simulink model "SP_linsysGet"  (R2016b)
settings: Solver=ode2  StartTime=0.0  StopTime=1  FixedStep=0.02  RelTol=1e-3
StopFcn:
  | A = StateSpace.A.Data(:,:,end);
  | B = StateSpace.B.Data(:,:,end);
  | C = StateSpace.C.Data(:,:,end);
  | if ( size(C,1) == 1 )
  |    D = StateSpace.D.Data(end);
  | else
  |    D = StateSpace.D.Data(:,:,end);
  | end
  | 
  | save linsys.mat A B C D;
undefined symbols (not defined in the file or in its folder): op
libraries: aerolibatmos2 x1
settings Model: Creator=whn  LastModifiedBy=whn
settings DataIOCC: SaveFormat=StructureWithTime
settings OptimizationCC: LifeSpan=inf
settings DebuggingCC: SFExecutionAtInitializationDiag=none
settings HardwareCC: ProdBitPerSizeT=32  ProdBitPerPtrDiffT=32  ProdWordSize=32  ProdHWDeviceType=Specified
settings ConfigComp: CovSFcnEnable=off

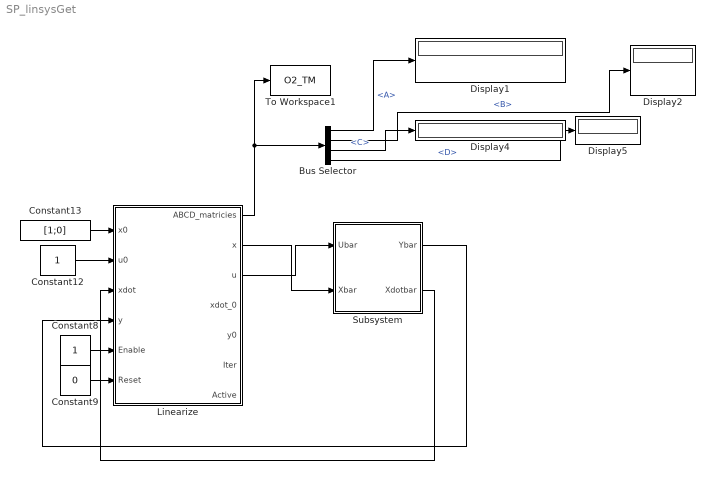
== system SP_linsysGet ==
  Bus Selector : BusSelector  OutputSignals=A,B,C,D
  Constant12 : Constant  VectorParams1D=off
  Constant13 : Constant  Value=[1;0]  VectorParams1D=off
  Constant8 : Constant
  Constant9 : Constant  Value=0
  Display{1..2,4..5} (4 alike) : Display
  Linearize : Subsystem  TreatAsAtomicUnit=on  mask(T-MATS: Linearize Library Block){N_XPer_M=[0.001 0.001], N_UPer_M=0.001, N_Y_M=1}
      mask prompts: N_XPer_M "N_XPer_M - x Perturbation values (mx1)"; N_UPer_M "N_UPer_M - u Perturbation values (nx1)"; N_Y_M "N_Y_M - Number of expected y values (1x1)"
      mask help:
      | Determine State-space equation for a given system where:
      |
      | (xdot - xdot_0) = A*(x - x0) + B*(u - u0)
      | (y - y0) = C*(x - x0) + D*(u - u0)
      |
      | During operation each plant state (x) and input (u) will be set to an initial condition then perturbed separately. Perturbed inputs and system effects are compared against the baseline to determine the A,B,C, and D matricies. Perturbation sized are specified below. x0, u0, xdot_0, and y0 values are initial conditions.
      | Matrix sizes are specified as:
      | xdot and x : mx1
      | y : px1
      | u : nx1
      | A : mxm
      | B : mxn
      | C : pxm
      | D : pxn
      mask Help: web(which('Solver_TMATS_Linearize.html'),'-helpbrowser')
  Subsystem : Subsystem
  To Workspace1 : ToWorkspace  VariableName=O2_TM  SaveFormat=Timeseries  SampleTime=-1
  wires:
  Constant8/1 -> Linearize/5(Enable)
  Constant9/1 -> Linearize/6(Reset)
  Constant12/1 -> Linearize/2(u0)
  Constant13/1 -> Linearize/1(x0)
  Bus Selector/1 -> Display1/1  "<A>"
  Bus Selector/2 -> Display2/1  "<B>"
  Bus Selector/3 -> Display4/1  "<C>"
  Bus Selector/4 -> Display5/1  "<D>"
  Linearize/1(ABCD_matricies) -> Bus Selector/1, To Workspace1/1
  Linearize/3(u) -> Subsystem/1(Ubar)
  Subsystem/1(Ybar) -> Linearize/4(y)
  Subsystem/2(Xdotbar) -> Linearize/3(xdot)
  Linearize/2(x) -> Subsystem/2(Xbar)

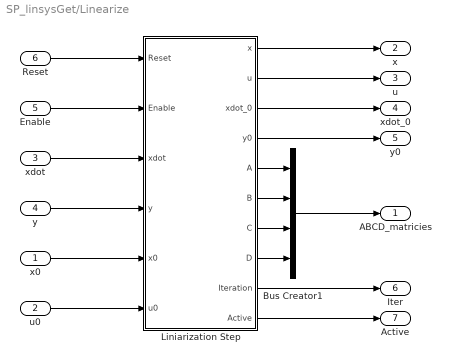
== system SP_linsysGet/Linearize ==
  x0 : Inport
  u0 : Inport  Port=2
  xdot : Inport  Port=3
  y : Inport  Port=4
  Enable : Inport  Port=5
  Reset : Inport  Port=6
  Bus Creator1 : BusCreator  Inputs=4
  Liniarization Step : Subsystem  TreatAsAtomicUnit=on
  ABCD_matricies : Outport
  x : Outport  Port=2
  u : Outport  Port=3
  xdot_0 : Outport  Port=4
  y0 : Outport  Port=5
  Iter : Outport  Port=6
  Active : Outport  Port=7
  wires:
  Enable/1 -> Liniarization Step/2(Enable)
  xdot/1 -> Liniarization Step/3(xdot)
  Bus Creator1/1 -> ABCD_matricies/1
  Reset/1 -> Liniarization Step/1(Reset)
  Liniarization Step/1(x) -> x/1
  Liniarization Step/2("u ") -> u/1
  Liniarization Step/5(A) -> Bus Creator1/1
  Liniarization Step/6(B) -> Bus Creator1/2
  Liniarization Step/7(C) -> Bus Creator1/3
  Liniarization Step/8(D) -> Bus Creator1/4
  y/1 -> Liniarization Step/4(y)
  x0/1 -> Liniarization Step/5(x0)
  u0/1 -> Liniarization Step/6(u0)
  Liniarization Step/9(Iteration) -> Iter/1
  Liniarization Step/10(Active) -> Active/1
  Liniarization Step/3(xdot_0) -> xdot_0/1
  Liniarization Step/4(y0) -> y0/1

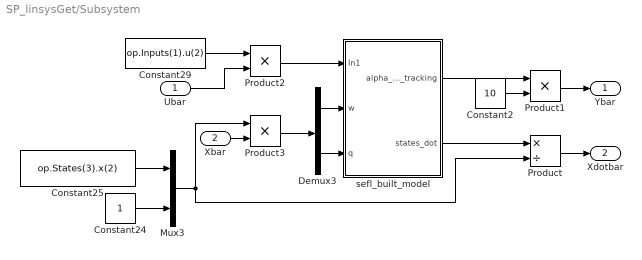
== system SP_linsysGet/Subsystem ==
  Ubar : Inport
  Xbar : Inport  Port=2
  Constant2 : Constant  Value=10
  Constant24 : Constant
  Constant25 : Constant  Value=op.States(3).x(2)
  Constant29 : Constant  Value=op.Inputs(1).u(2)
  Demux3 : Demux  Outputs=2
  Mux3 : Mux  Inputs=2
  Product : Product  Inputs=*/
  Product1 : Product
  Product2 : Product
  Product3 : Product
  sefl_built_model : Subsystem
  Ybar : Outport
  Xdotbar : Outport  Port=2
  wires:
  Mux3/1 -> Product/2, Product3/1
  Xbar/1 -> Product3/2
  sefl_built_model/1(alpha_for_tracking) -> Product1/1
  Product1/1 -> Ybar/1
  Product3/1 -> Demux3/1
  sefl_built_model/2(states_dot) -> Product/1
  Constant29/1 -> Product2/1
  Constant2/1 -> Product1/2
  Product2/1 -> sefl_built_model/1(In1)
  Product/1 -> Xdotbar/1
  Demux3/1 -> sefl_built_model/2(w)
  Constant25/1 -> Mux3/1
  Constant24/1 -> Mux3/2
  Demux3/2 -> sefl_built_model/3(q)
  Ubar/1 -> Product2/2

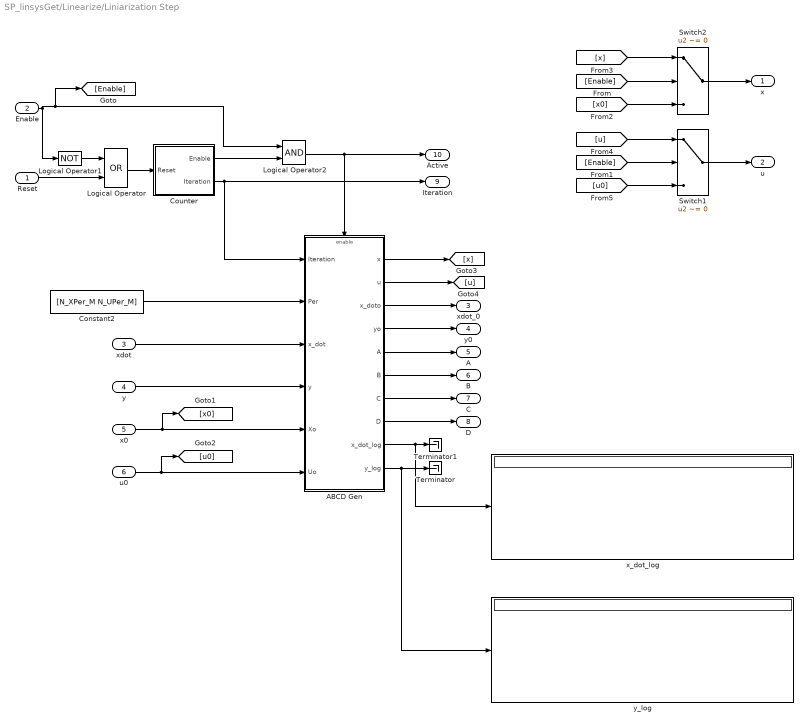
== system SP_linsysGet/Linearize/Liniarization Step ==
  Reset : Inport
  Enable : Inport  Port=2
  xdot : Inport  Port=3
  y : Inport  Port=4
  x0 : Inport  Port=5
  u0 : Inport  Port=6
  ABCD Gen : Subsystem
  Constant2 : Constant  Value=[N_XPer_M N_UPer_M]
  Counter : Subsystem  mask{N_Ind_M=length(N_XPer_M) + length(N_UPer_M)}
      mask prompts: N_Ind_M "number of independents, N_Ind_M"
  Logical Operator : Logic  Operator=OR  AllPortsSameDT=off  OutDataTypeStr=boolean
  Logical Operator1 : Logic  Operator=NOT  AllPortsSameDT=off  OutDataTypeStr=boolean
  Logical Operator2 : Logic  AllPortsSameDT=off  OutDataTypeStr=boolean
  Switch1 : Switch  Criteria=u2 ~= 0
  Switch2 : Switch  Criteria=u2 ~= 0
  Terminator : Terminator
  Terminator1 : Terminator
  x_dot_log : Display
  y_log : Display
  x : Outport
  "u " : Outport  Port=2
  xdot_0 : Outport  Port=3
  y0 : Outport  Port=4
  A : Outport  Port=5
  B : Outport  Port=6
  C : Outport  Port=7
  D : Outport  Port=8
  Iteration : Outport  Port=9
  Active : Outport  Port=10
  wires:
  [x] -> Switch2/1
  [x0] -> Switch2/3
  [u0] -> Switch1/3
  [u] -> Switch1/1
  Switch1/1 -> "u "/1
  Switch2/1 -> x/1
  [Enable] -> Switch1/2
  [Enable] -> Switch2/2
  Enable/1 -> Logical Operator1/1, Logical Operator2/1, [Enable]
  Counter/1(Enable) -> Logical Operator2/2
  Logical Operator1/1 -> Logical Operator/1
  Logical Operator/1 -> Counter/1(Reset)
  ABCD Gen/7(C) -> C/1
  ABCD Gen/8(D) -> D/1
  Counter/2(Iteration) -> ABCD Gen/1(Iteration), Iteration/1
  x0/1 -> ABCD Gen/5(Xo), [x0]
  Logical Operator2/1 -> Active/1, ABCD Gen/Enable
  Reset/1 -> Logical Operator/2
  ABCD Gen/1(x) -> [x]
  Constant2/1 -> ABCD Gen/2(Per)
  xdot/1 -> ABCD Gen/3(x_dot)
  u0/1 -> ABCD Gen/6(Uo), [u0]
  y/1 -> ABCD Gen/4(y)
  ABCD Gen/10(y_log) -> y_log/1, Terminator/1
  ABCD Gen/9(x_dot_log) -> x_dot_log/1, Terminator1/1
  ABCD Gen/2(u) -> [u]
  ABCD Gen/5(A) -> A/1
  ABCD Gen/6(B) -> B/1
  ABCD Gen/3(x_doto) -> xdot_0/1
  ABCD Gen/4(yo) -> y0/1

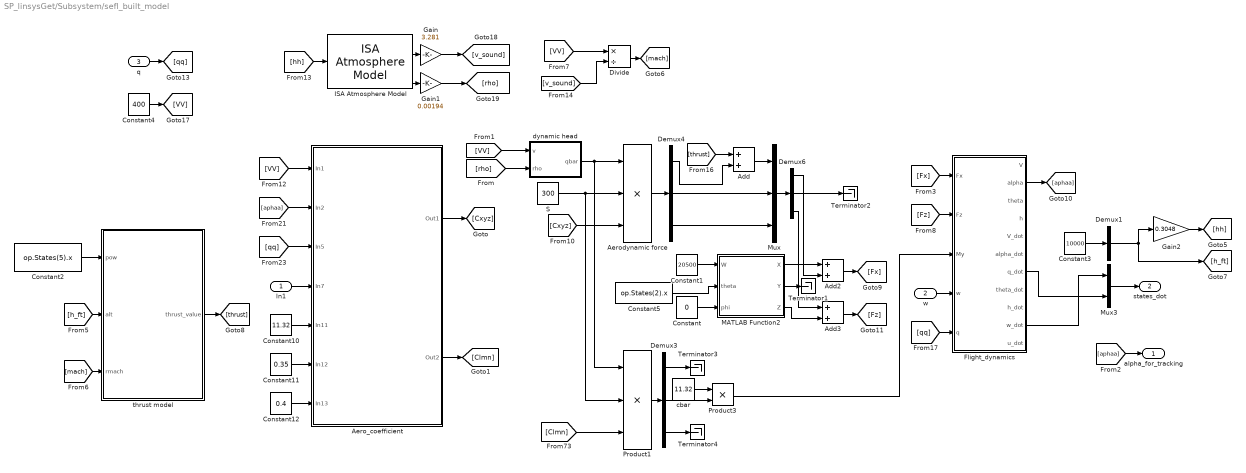
== system SP_linsysGet/Subsystem/sefl_built_model ==
  In1 : Inport
  w : Inport  Port=2
  q : Inport  Port=3
  Add : Sum
  Add2 : Sum
  Add3 : Sum
  Aero_coefficient : Subsystem
      mask Display:
      | port_label('input', 1, 'vt')
      | port_label('input', 2, 'alpha')
      | 
      | port_label('input', 3, 'q')
      | 
      | port_label('input', 4, 'el')
      | 
      | 
      | 
      | port_label('input', 5, 'cbar')
      | port_label('input', 6, 'xcgr')
      | port_label('input', 7, 'xcg')
      | port_label('output', 1, 'Cxz')
      | port_label('output', 2, 'Cm')
  "Aerodynamic force " : Product  Inputs=3
  Constant : Constant  Value=0
  Constant1 : Constant  Value=20500
  Constant10 : Constant  Value=11.32
  Constant11 : Constant  Value=0.35
  Constant12 : Constant  Value=0.4
  Constant2 : Constant  Value=op.States(5).x
  Constant3 : Constant  Value=10000
  Constant4 : Constant  Value=400
  Constant5 : Constant  Value=op.States(2).x
  Demux1 : Demux  Outputs=1
  Demux3 : Demux  Outputs=3
  Demux4 : Demux  Outputs=3
  Demux6 : Demux  Outputs=3
  Divide : Product  Inputs=*/
  Flight_dynamics : Subsystem
  Gain : Gain  Gain=3.281
  Gain1 : Gain  Gain=0.00194
  Gain2 : Gain  Gain=0.3048
  ISA Atmosphere Model : aerolibatmos2/ISA Atmosphere Model  custom=off  g=9.80665  gamma=1.4  R=287.0531  L=0.0065  h_trop=11000  h_strat=20000  rho0=1.225  P0=101325  T0=288.15  h0=0
  MATLAB Function2 : MATLAB Function  TreatAsAtomicUnit=on
  Mux : Mux  Inputs=3
  Mux3 : Mux  Inputs=2
  Product1 : Product  Inputs=3
  Product3 : Product
  S : Constant  Value=300
  Terminator{1..4} (4 alike) : Terminator
  cbar : Constant  Value=11.32
  dynamic head : MATLAB Function  TreatAsAtomicUnit=on
  thrust model : MATLAB Function  TreatAsAtomicUnit=on
  alpha_for_tracking : Outport
  states_dot : Outport  Port=2
  wires:
  Flight_dynamics/2(alpha) -> [aphaa]
  Mux3/1 -> states_dot/1
  Product3/1 -> Flight_dynamics/3(My)
  [Fz] -> Flight_dynamics/2(Fz)
  [Fx] -> Flight_dynamics/1(Fx)
  Add3/1 -> [Fz]
  Add2/1 -> [Fx]
  MATLAB Function2/2(Y) -> Terminator1/1
  MATLAB Function2/3(Z) -> Add3/2
  Demux6/1 -> Add2/2
  MATLAB Function2/1(X) -> Add2/1
  Constant/1 -> MATLAB Function2/3(phi)
  Constant5/1 -> MATLAB Function2/2(theta)
  Constant1/1 -> MATLAB Function2/1(W)
  Demux6/2 -> Terminator2/1
  Demux6/3 -> Add3/1
  cbar/1 -> Product3/1
  Demux3/2 -> Product3/2
  Product1/1 -> Demux3/1
  [Clmn] -> Product1/3
  S/1 -> Product1/2, "Aerodynamic force "/2
  [Cxyz] -> "Aerodynamic force "/3
  "Aerodynamic force "/1 -> Demux4/1
  [thrust] -> Add/1
  [mach] -> thrust model/3(rmach)
  [h_ft] -> thrust model/2(alt)
  thrust model/1(thrust_value) -> [thrust]
  Gain2/1 -> [hh]
  Constant12/1 -> Aero_coefficient/7(In13)
  Mux/1 -> Demux6/1
  Demux4/1 -> Add/2
  [v_sound] -> Divide/2
  Demux4/2 -> Mux/2
  Add/1 -> Mux/1
  Divide/1 -> [mach]
  Gain/1 -> [v_sound]
  Demux4/3 -> Mux/3
  [hh] -> ISA Atmosphere Model/1
  Demux1/1 -> [h_ft], Gain2/1
  Aero_coefficient/2(Out2) -> [Clmn]
  [rho] -> dynamic head/2(rho)
  Aero_coefficient/1(Out1) -> [Cxyz]
  [VV] -> dynamic head/1(v)
  [VV] -> Divide/1
  Gain1/1 -> [rho]
  Constant11/1 -> Aero_coefficient/6(In12)
  Constant10/1 -> Aero_coefficient/5(In11)
  In1/1 -> Aero_coefficient/4(In7)
  dynamic head/1(qbar) -> "Aerodynamic force "/1, Product1/1
  ISA Atmosphere Model/2 -> Gain/1
  ISA Atmosphere Model/4 -> Gain1/1
  [VV] -> Aero_coefficient/1(In1)
  [aphaa] -> Aero_coefficient/2(In2)
  [qq] -> Aero_coefficient/3(In5)
  q/1 -> [qq]
  Flight_dynamics/10(w_dot) -> Mux3/1
  Flight_dynamics/7(q_dot) -> Mux3/2
  Constant2/1 -> thrust model/1(pow)
  Constant3/1 -> Demux1/1
  Constant4/1 -> [VV]
  [aphaa] -> alpha_for_tracking/1
  w/1 -> Flight_dynamics/4(w)
  [qq] -> Flight_dynamics/5(q)
  Demux3/1 -> Terminator3/1
  Demux3/3 -> Terminator4/1

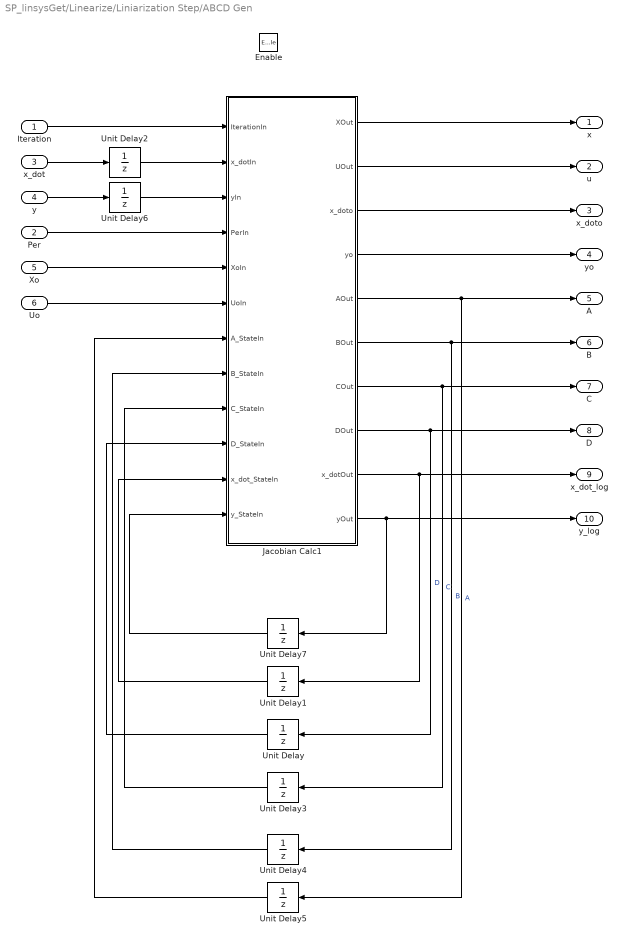
== system SP_linsysGet/Linearize/Liniarization Step/ABCD Gen ==
  Iteration : Inport
  Per : Inport  Port=2
  x_dot : Inport  Port=3
  y : Inport  Port=4
  Xo : Inport  Port=5
  Uo : Inport  Port=6
  Enable : EnablePort
  Jacobian Calc1 : MATLAB Function  TreatAsAtomicUnit=on
  Unit Delay : UnitDelay  InitialCondition=zeros(N_Y_M,length(N_UPer_M))  SampleTime=-1
  Unit Delay1 : UnitDelay  InitialCondition=zeros(length(N_XPer_M),length(N_XPer_M)+length(N_UPer_M)+1)  SampleTime=-1
  Unit Delay2 : UnitDelay  InitialCondition=zeros(length(N_XPer_M),1)  SampleTime=-1
  Unit Delay3 : UnitDelay  InitialCondition=zeros(N_Y_M,length(N_XPer_M))  SampleTime=-1
  Unit Delay4 : UnitDelay  InitialCondition=zeros(length(N_XPer_M),length(N_UPer_M))  SampleTime=-1
  Unit Delay5 : UnitDelay  InitialCondition=zeros(length(N_XPer_M),length(N_XPer_M))  SampleTime=-1
  Unit Delay6 : UnitDelay  InitialCondition=zeros(length(N_Y_M),1)  SampleTime=-1
  Unit Delay7 : UnitDelay  InitialCondition=zeros(N_Y_M,length(N_XPer_M)+length(N_UPer_M)+1)  SampleTime=-1
  x : Outport
  u : Outport  Port=2
  x_doto : Outport  Port=3
  yo : Outport  Port=4
  A : Outport  Port=5
  B : Outport  Port=6
  C : Outport  Port=7
  D : Outport  Port=8
  x_dot_log : Outport  Port=9
  y_log : Outport  Port=10
  wires:
  Unit Delay2/1 -> Jacobian Calc1/2(x_dotIn)
  x_dot/1 -> Unit Delay2/1
  Unit Delay1/1 -> Jacobian Calc1/11(x_dot_StateIn)
  Jacobian Calc1/9(x_dotOut) -> Unit Delay1/1, x_dot_log/1
  Jacobian Calc1/8(DOut) -> Unit Delay/1, D/1  "D"
  Jacobian Calc1/7(COut) -> Unit Delay3/1, C/1  "C"
  Iteration/1 -> Jacobian Calc1/1(IterationIn)
  Per/1 -> Jacobian Calc1/4(PerIn)
  Xo/1 -> Jacobian Calc1/5(XoIn)
  Jacobian Calc1/1(XOut) -> x/1
  Jacobian Calc1/6(BOut) -> Unit Delay4/1, B/1  "B"
  Jacobian Calc1/5(AOut) -> Unit Delay5/1, A/1  "A"
  Unit Delay/1 -> Jacobian Calc1/10(D_StateIn)
  Unit Delay3/1 -> Jacobian Calc1/9(C_StateIn)
  Unit Delay4/1 -> Jacobian Calc1/8(B_StateIn)
  Unit Delay5/1 -> Jacobian Calc1/7(A_StateIn)
  Uo/1 -> Jacobian Calc1/6(UoIn)
  Jacobian Calc1/2(UOut) -> u/1
  Jacobian Calc1/10(yOut) -> Unit Delay7/1, y_log/1
  Unit Delay6/1 -> Jacobian Calc1/3(yIn)
  y/1 -> Unit Delay6/1
  Unit Delay7/1 -> Jacobian Calc1/12(y_StateIn)
  Jacobian Calc1/3(x_doto) -> x_doto/1
  Jacobian Calc1/4(yo) -> yo/1

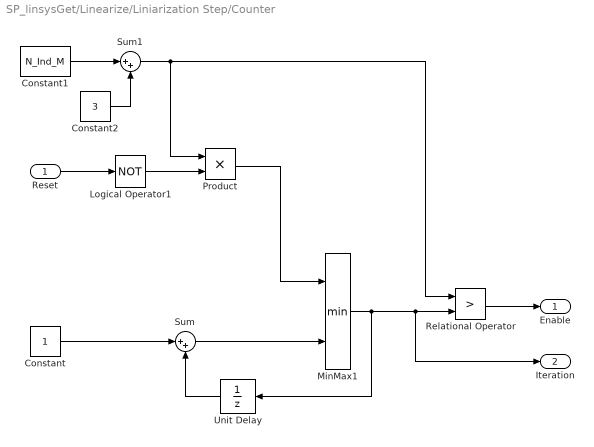
== system SP_linsysGet/Linearize/Liniarization Step/Counter ==
  Reset : Inport
  Constant : Constant
  Constant1 : Constant  Value=N_Ind_M
  Constant2 : Constant  Value=3
  Logical Operator1 : Logic  Operator=NOT  AllPortsSameDT=off  OutDataTypeStr=boolean
  MinMax1 : MinMax  Inputs=2
  Product : Product  RndMeth=Zero
  Relational Operator : RelationalOperator  Operator=>  OutDataTypeStr=boolean  RndMeth=Nearest
  Sum : Sum  Inputs=|++
  Sum1 : Sum  Inputs=|++
  Unit Delay : UnitDelay  SampleTime=-1
  Enable : Outport
  Iteration : Outport  Port=2
  wires:
  Constant1/1 -> Sum1/1
  Constant2/1 -> Sum1/2
  Sum1/1 -> Product/1, Relational Operator/1
  Reset/1 -> Logical Operator1/1
  Logical Operator1/1 -> Product/2
  Relational Operator/1 -> Enable/1
  MinMax1/1 -> Relational Operator/2, Iteration/1, Unit Delay/1
  Unit Delay/1 -> Sum/2
  Sum/1 -> MinMax1/2
  Product/1 -> MinMax1/1
  Constant/1 -> Sum/1

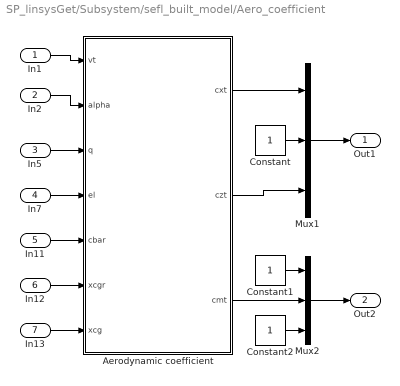
== system SP_linsysGet/Subsystem/sefl_built_model/Aero_coefficient ==
  In1 : Inport
  In2 : Inport  Port=2
  In5 : Inport  Port=3
  In7 : Inport  Port=4
  In11 : Inport  Port=5
  In12 : Inport  Port=6
  In13 : Inport  Port=7
  Aerodynamic coefficient : MATLAB Function  TreatAsAtomicUnit=on
  Constant : Constant
  Constant1 : Constant
  Constant2 : Constant
  Mux1 : Mux  Inputs=3
  Mux2 : Mux  Inputs=3
  Out1 : Outport
  Out2 : Outport  Port=2
  wires:
  Constant2/1 -> Mux2/3
  Constant1/1 -> Mux2/1
  Constant/1 -> Mux1/2
  Mux2/1 -> Out2/1
  Mux1/1 -> Out1/1
  Aerodynamic coefficient/1(cxt) -> Mux1/1
  In13/1 -> Aerodynamic coefficient/7(xcg)
  Aerodynamic coefficient/2(czt) -> Mux1/3
  In12/1 -> Aerodynamic coefficient/6(xcgr)
  In11/1 -> Aerodynamic coefficient/5(cbar)
  Aerodynamic coefficient/3(cmt) -> Mux2/2
  In7/1 -> Aerodynamic coefficient/4(el)
  In2/1 -> Aerodynamic coefficient/2(alpha)
  In1/1 -> Aerodynamic coefficient/1(vt)
  In5/1 -> Aerodynamic coefficient/3(q)

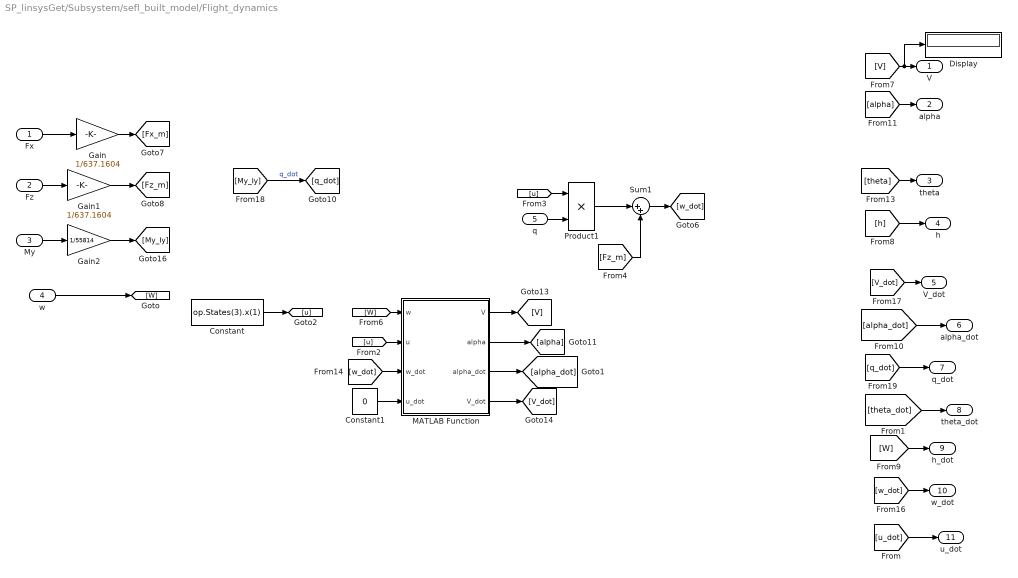
== system SP_linsysGet/Subsystem/sefl_built_model/Flight_dynamics ==
  Fx : Inport
  Fz : Inport  Port=2
  My : Inport  Port=3
  w : Inport  Port=4
  q : Inport  Port=5
  Constant : Constant  Value=op.States(3).x(1)
  Constant1 : Constant  Value=0
  Display : Display
  Gain : Gain  Gain=1/637.1604
  Gain1 : Gain  Gain=1/637.1604
  Gain2 : Gain  Gain=1/55814
  MATLAB Function : MATLAB Function  TreatAsAtomicUnit=on
  Product1 : Product
  Sum1 : Sum  Inputs=|++
  V : Outport
  alpha : Outport  Port=2
  theta : Outport  Port=3
  h : Outport  Port=4
  V_dot : Outport  Port=5
  alpha_dot : Outport  Port=6
  q_dot : Outport  Port=7
  theta_dot : Outport  Port=8
  h_dot : Outport  Port=9
  w_dot : Outport  Port=10
  u_dot : Outport  Port=11
  wires:
  [u_dot] -> u_dot/1
  [w_dot] -> w_dot/1
  [u] -> MATLAB Function/2(u)
  [W] -> h_dot/1
  [h] -> h/1
  MATLAB Function/4(V_dot) -> [V_dot]
  MATLAB Function/1(V) -> [V]
  [theta_dot] -> theta_dot/1
  [q_dot] -> q_dot/1
  [alpha_dot] -> alpha_dot/1
  [V_dot] -> V_dot/1
  [theta] -> theta/1
  [alpha] -> alpha/1
  [V] -> V/1, Display/1
  MATLAB Function/3(alpha_dot) -> [alpha_dot]
  [w_dot] -> MATLAB Function/3(w_dot)
  MATLAB Function/2(alpha) -> [alpha]
  [W] -> MATLAB Function/1(w)
  [My_Iy] -> [q_dot]  "q_dot"
  Sum1/1 -> [w_dot]
  [Fz_m] -> Sum1/2
  Product1/1 -> Sum1/1
  Gain2/1 -> [My_Iy]
  My/1 -> Gain2/1
  Gain1/1 -> [Fz_m]
  Gain/1 -> [Fx_m]
  Fz/1 -> Gain1/1
  Fx/1 -> Gain/1
  Constant/1 -> [u]
  Constant1/1 -> MATLAB Function/4(u_dot)
  [u] -> Product1/1
  w/1 -> [W]
  q/1 -> Product1/2

== matlab function SP_linsysGet/Linearize/Liniarization Step/ABCD Gen/Jacobian Calc1 ==
  data: IterationIn input; XOut output; x_dotIn input; yIn input; PerIn input; XoIn input; UoIn input; A_StateIn input size=[length(N_XPer_M) length(N_XPer_M)]; B_StateIn input size=[length(N_XPer_M) length(N_UPer_M)]; C_StateIn input size=[N_Y_M length(N_XPer_M)]; D_StateIn input size=[N_Y_M length(N_UPer_M)]; x_dot_StateIn input; UOut output; x_doto output; yo output; AOut output; BOut output; COut output size=[N_Y_M length(N_XPer_M)]; DOut output; x_dotOut output; yOut output; y_StateIn input size=[N_Y_M,length(N_XPer_M)+length(N_UPer_M)+1]
function [ XOut, UOut, x_doto, yo, AOut, BOut, COut, DOut, x_dotOut, yOut ] = fcn ...
( IterationIn, x_dotIn, yIn, PerIn, XoIn, UoIn, A_StateIn, B_StateIn, C_StateIn, D_StateIn, x_dot_StateIn, y_StateIn )

% Set inital condiations
i = IterationIn;
XOut = XoIn;
UOut = UoIn;
AOut = A_StateIn;
BOut = B_StateIn;
COut = C_StateIn;
DOut = D_StateIn;
x_dotOut = x_dot_StateIn;
yOut = y_StateIn;

x_doto = x_dot_StateIn(:,1);
yo = y_StateIn(:,1);

% Begin taking data from f(x) at iteration a+1
a = 1;
% Begin determining Jacobian at iteration b+1
b = a+1;
c = a+length(XoIn);
d = c+1;

% Set X&U Output
if i > a && i <= length(XoIn) + a
    XOut(i-a) = XOut(i-a) + PerIn(i - a);
elseif i > c && i <= length(UoIn) + c
    UOut(i-c) = UOut(i-c) + PerIn(i - a);
end

% setup state feedback
if i > a && i<= length(XoIn) + length(UoIn) + a+1;
        x_dotOut(:,i - a) = x_dotIn;
        yOut(:,i - a) = yIn;
end

% Create Jacobian
if i > b && i <= length(XoIn) + b
    if length(XoIn) == 1
        AOut = (x_dotIn - x_dotOut(:,1))/PerIn(1);
        COut = (yIn - yOut(:,1))/PerIn(1);
    else
        AOut(:,i - b) = (x_dotIn - x_dotOut(:,1))/PerIn(i - b);
        COut(:,i - b) = (yIn - yOut(:,1))/PerIn(i - b);
    end
end
if i > d && i <= length(UoIn) + d
    if length(UoIn) == 1
        BOut = (x_dotIn - x_dotOut(:,1))/PerIn(c);
        DOut = (yIn - yOut(:,1))/PerIn(c);
    else
        BOut(:,i - d) = (x_dotIn - x_dotOut(:,1))/PerIn(i - d);
        DOut(:,i - d) = (yIn - yOut(:,1))/PerIn(i - d);
    end
end

== matlab function SP_linsysGet/Subsystem/sefl_built_model/Aero_coefficient/Aerodynamic coefficient ==
  data: vt input; alpha input; q input; cxt output; el input; czt output; cmt output; cbar input; xcgr input; xcg input
function [cxt,czt,cmt]=fcn(vt,alpha,q,el,cbar,xcgr,xcg)
%% ---- Look-up tables and component biuldup ------------
beta=0;
rtod = 180 / pi;
alpha=alpha*rtod;
beta=beta*rtod;
% el=el*rtod;
% ail=ail*rtod;
% rdr=rdr*rtod;
cxt = cx ( alpha, el );
%cyt = cy ( beta, ail, rdr );
czt = cz ( alpha, beta, el );
%dail = ail / 20.0;
%drdr = rdr / 30.0;
%dlda_value = dlda( alpha, beta );
%dldr_value = dldr( alpha, beta );
%clt = cl( alpha, beta ) + dlda_value * dail + dldr_value * drdr;
cmt = cm( alpha, el );
%dnda_value = dnda( alpha, beta );
%dndr_value = dndr( alpha, beta );
%cnt = cn( alpha, beta ) + dnda_value * dail + dndr_value * drdr;

%% ---- Add damping derivatives ------------
tvt = 0.5 / vt;
%b2v = b * tvt;
cq = cbar * q * tvt;
d = damping( alpha );
cxt = cxt + cq * d(1);
%cyt = cyt + b2v * ( d(2) * r + d(3) * p );
czt = czt + cq * d(4);
%clt = clt + b2v * ( d(5) * r + d(6) * p );
cmt = cmt + cq * d(7) + czt * ( xcgr - xcg );
%cnt = cnt + b2v * ( d(8)* r + d(9) * p ) - cyt * ( xcgr - xcg ) * cbar / b;

function dlda_value = dlda ( alpha, beta )

A = [ -.041  -.052  -.053  -.056  -.050  -.056  -.082  -.059  -.042  -.038  -.027  -.017;
      -.041  -.053  -.053  -.053  -.050  -.051  -.066  -.043  -.038  -.027  -.023  -.016;
      -.042  -.053  -.052  -.051  -.049  -.049  -.043  -.035  -.026  -.016  -.018  -.014;
      -.040  -.052  -.051  -.052  -.048  -.048  -.042  -.037  -.031  -.026  -.017  -.012;
      -.043  -.049  -.048  -.049  -.043  -.042  -.042  -.036  -.025  -.021  -.016  -.011;
      -.044  -.048  -.048  -.047  -.042  -.041  -.020  -.028  -.013  -.014  -.011  -.010;
      -.043  -.049  -.047  -.045  -.042  -.037  -.003  -.013  -.010  -.003  -.007  -.008 ];
A = A';  
row = 3;
col = 4;

s = 0.2 * alpha;
k = fix ( s );
if ( k <= -2 )
    k = -1;
end
if ( k >= 9 )
    k = 8;
end
da = s -  k ;
l = k + fix ( sign ( da ) * 1.1 );
%%%%%%%%%%%%%%%%%%%%%%%%%%%%%%%%%%
% added as boundary condition
if l < -2
    l = -2;
elseif l > 9
        l = 9;
end
%%%%%%%%%%%%%%%%%%%%%%%%%%%%%%%%%%
s = 0.1 * beta;
m = fix ( s );
if ( m <= -3 )
   m = -2;
end
if ( m >= 3)
   m = 2;
end
db = s -  m ;
n = m + fix ( sign ( db ) * 1.1 );
%%%%%%%%%%%%%%%%%%%%%%%%%%%%%%%%%%
% added as boundary condition
if n < -3
    n = -3;
elseif n > 3
        n = 3;
end
%%%%%%%%%%%%%%%%%%%%%%%%%%%%%%%%%%
%  disp('k+row'); k+row
%  disp('m+col'); m+col
%  disp('n+col'); n+col
%  disp('l+row'); l+row
t = A( k+row, m+col );
u = A( k+row, n+col );
v = t + abs( da ) * ( A( l+row, m+col ) - t );
w = u + abs( da ) * ( A( l+row, n+col ) - u );
dlda_value = v + ( w - v ) * abs( db );

function dldr_value = dldr ( alpha, beta )

A = [ .005  .017  .014  .010  -.005  .009  .019  .005   .000  -.005  -.011  .008;
      .007  .016  .014  .014   .013  .009  .012  .005   .000   .004   .009  .007;
      .013  .013  .011  .012   .011  .009  .008  .005   .000   .005   .003  .005;
      .018  .015  .015  .014   .014  .014  .014  .015   .013   .011   .006  .001;
      .015  .014  .013  .013   .012  .011  .011  .010   .008   .008   .007  .003;
      .021  .011  .010  .011   .010  .009  .008  .010   .006   .005   .000  .001;
      .023  .010  .011  .011   .011  .010  .008  .010   .006   .014   .020  .000 ];
A = A';  
row = 3;
col = 4;

s = 0.2 * alpha;
k = fix ( s );
if ( k <= -2 )
    k = -1;
end
if ( k >= 9 )
    k = 8;
end
da = s -  k ;
l = k + fix ( sign ( da ) * 1.1 );
%%%%%%%%%%%%%%%%%%%%%%%%%%%%%%%%%%
% added as boundary condition
if l < -2
    l = -2;
elseif l > 9
        l = 9;
end
%%%%%%%%%%%%%%%%%%%%%%%%%%%%%%%%%%
s = 0.1 * beta;
m = fix ( s );
if ( m <= -3 )
   m = -2;
end
if ( m >= 3)
   m = 2;
end
db = s -  m ;
n = m + fix ( sign ( db ) * 1.1 );
%%%%%%%%%%%%%%%%%%%%%%%%%%%%%%%%%%
% added as boundary condition
if n < -3
    n = -3;
elseif n > 3
        n = 3;
end
%%%%%%%%%%%%%%%%%%%%%%%%%%%%%%%%%%
t = A( k+row, m+col );
u = A( k+row, n+col );
v = t + abs( da ) * ( A( l+row, m+col ) - t );
w = u + abs( da ) * ( A( l+row, n+col ) - u );
dldr_value = v + ( w - v ) * abs( db );

function dnda_value = dnda ( alpha, beta )

A = [  .001  -.027  -.017  -.013  -.012  -.016   .001   .017   .011  .017   .008  .016
       .002  -.014  -.016  -.016  -.014  -.019  -.021   .002   .012  .016   .015  .011
      -.006  -.008  -.006  -.006  -.005  -.008  -.005   .007   .004  .007   .006  .006
      -.011  -.011  -.010  -.009  -.008  -.006   .000   .004   .007  .010   .004  .010
      -.015  -.015  -.014  -.012  -.011  -.008  -.002   .002   .006  .012   .011  .011
      -.024  -.010  -.004  -.002  -.001   .003   .014   .006  -.001  .004   .004  .006
      -.022   .002  -.003  -.005  -.003  -.001  -.009  -.009  -.001  .003  -.002  .001  ];
A = A';  
row = 3;
col = 4;

s = 0.2 * alpha;
k = fix ( s );
if ( k <= -2 )
    k = -1;
end
if ( k >= 9 )
    k = 8;
end
da = s -  k ;
l = k + fix ( sign ( da ) * 1.1 );
%%%%%%%%%%%%%%%%%%%%%%%%%%%%%%%%%%
% added as boundary condition
if l < -2
    l = -2;
elseif l > 9
        l = 9;
end
%%%%%%%%%%%%%%%%%%%%%%%%%%%%%%%%%%
s = 0.1 * beta;
m = fix ( s );
if ( m <= -3 )
   m = -2;
end
if ( m >= 3)
   m = 2;
end
db = s -  m ;
n = m + fix ( sign ( db ) * 1.1 );
%%%%%%%%%%%%%%%%%%%%%%%%%%%%%%%%%%
% added as boundary condition
if n < -3
    n = -3;
elseif n > 3
        n = 3;
end
%%%%%%%%%%%%%%%%%%%%%%%%%%%%%%%%%%
t = A( k+row, m+col );
u = A( k+row, n+col );
v = t + abs( da ) * ( A( l+row, m+col ) - t );
w = u + abs( da ) * ( A( l+row, n+col ) - u );
dnda_value = v + ( w - v ) * abs( db );

function dndr_value = dndr ( alpha, beta )

A = [ -.018  -.052  -.052  -.052  -.054  -.049  -.059  -.051  -.030  -.037  -.026  -.013;
      -.028  -.051  -.043  -.046  -.045  -.049  -.057  -.052  -.030  -.033  -.030  -.008;
      -.037  -.041  -.038  -.040  -.040  -.038  -.037  -.030  -.027  -.024  -.019  -.013; 
      -.048  -.045  -.045  -.045  -.044  -.045  -.047  -.048  -.049  -.045  -.033  -.016;
      -.043  -.044  -.041  -.041  -.040  -.038  -.034  -.035  -.035  -.029  -.022  -.009;
      -.052  -.034  -.036  -.036  -.035  -.028  -.024  -.023  -.020  -.016  -.010  -.014;
      -.062  -.034  -.027  -.028  -.027  -.027  -.023  -.023  -.019  -.009  -.025  -.010 ];
A = A';  
row = 3;
col = 4;

s = 0.2 * alpha;
k = fix ( s );
if ( k <= -2 )
    k = -1;
end
if ( k >= 9 )
    k = 8;
end
da = s -  k ;
l = k + fix ( sign ( da ) * 1.1 );
%%%%%%%%%%%%%%%%%%%%%%%%%%%%%%%%%%
% added as boundary condition
if l < -2
    l = -2;
elseif l > 9
        l = 9;
end
%%%%%%%%%%%%%%%%%%%%%%%%%%%%%%%%%%
s = 0.1 * beta;
m = fix ( s );
if ( m <= -3 )
   m = -2;
end
if ( m >= 3)
   m = 2;
end
db = s -  m ;
n = m + fix ( sign ( db ) * 1.1 );
%%%%%%%%%%%%%%%%%%%%%%%%%%%%%%%%%%
% added as boundary condition
if n < -3
    n = -3;
elseif n > 3
        n = 3;
end
%%%%%%%%%%%%%%%%%%%%%%%%%%%%%%%%%%
t = A( k+row, m+col );
u = A( k+row, n+col );
v = t + abs( da ) * ( A( l+row, m+col ) - t );
w = u + abs( da ) * ( A( l+row, n+col ) - u );
dndr_value = v + ( w - v ) * abs( db );

function cx_value = cx( alpha, el )

A = [ -0.099  -0.081  -0.081  -0.063  -0.025  0.044  0.097  0.113  0.145  0.167  0.174  0.166;
      -0.048  -0.038  -0.040  -0.021   0.016  0.083  0.127  0.137  0.162  0.177  0.179  0.167;
      -0.022  -0.020  -0.021  -0.004   0.032  0.094  0.128  0.130  0.154  0.161  0.155  0.138;
      -0.040  -0.038  -0.039  -0.025   0.006  0.062  0.087  0.085  0.100  0.110  0.104  0.091;
      -0.083  -0.073  -0.076  -0.072  -0.046  0.012  0.024  0.025  0.043  0.053  0.047  0.040 ];
A = A';  
row = 3;
col = 3;

s = 0.2 * alpha;
k = fix ( s );
if ( k <= -2 )
    k = -1;
end
if ( k >= 9 )
    k = 8;
end
da = s - k;
l = k + fix ( sign ( da ) * 1.1 );
%%%%%%%%%%%%%%%%%%%%%%%%%%%%%%%%%%
% added as boundary condition
if l < -2
    l = -2;
elseif l > 9
        l = 9;
end
%%%%%%%%%%%%%%%%%%%%%%%%%%%%%%%%%%
s = el / 12.0;
m = fix ( s );
if ( m <= -2 )
   m = -1;
end
if ( m >= 2)
   m = 1;
end
de = s - m;
n = m + fix ( sign ( de ) * 1.1 );
%%%%%%%%%%%%%%%%%%%%%%%%%%%%%%%%%%
% added as boundary condition
if n < -2
    n = -2;
elseif n > 2
        n = 2;
end
%%%%%%%%%%%%%%%%%%%%%%%%%%%%%%%%%%
t = A( k+row, m+col );
u = A( k+row, n+col );
v = t + abs( da ) * ( A( l+row, m+col ) - t );
w = u + abs( da ) * ( A( l+row, n+col ) - u );
cx_value = v + ( w - v ) * abs( de );

function cy_value = cy( beta, ail, rdr )

cy_value = -0.02 * beta + 0.021 * ( ail / 20.0 )+...
           0.086 * ( rdr / 30.0 );
       
function cz_value = cz( alpha, beta, el )

A = [ 0.770  0.241  -0.100  -0.416  -0.731  -1.053  -1.366  -1.646  -1.917  -2.120  -2.248  -2.229 ];
A = A';  
row = 3;

s = 0.2 * alpha;
k = fix ( s );
if ( k <= -2 )
    k = -1;
end
if ( k >= 9 )
    k = 8;
end
da = s - k;
l = k + fix ( sign ( da ) * 1.1 );
%%%%%%%%%%%%%%%%%%%%%%%%%%%%%%%%%%
% added as boundary condition
if l < -2
    l = -2;
elseif l > 9
        l = 9;
end
%%%%%%%%%%%%%%%%%%%%%%%%%%%%%%%%%%
s = A( k+row ) + abs( da ) * ( A( l+row ) - A( k+row ) );
cz_value = s * ( 1 - ( beta / 57.3 ) ^ 2 ) - 0.19 * ( el / 25.0 );

function cl_value = cl( alpha, beta )

A = [  .0     .0     .0     .0     .0     .0     .0     .0     .0     .0     .0     .0  ;
      -.001  -.004  -.008  -.012  -.016  -.022  -.022  -.021  -.015  -.008  -.013  -.015;
      -.003  -.009  -.017  -.024  -.030  -.041  -.045  -.040  -.016  -.002  -.010  -.019;
      -.001  -.010  -.020  -.030  -.039  -.054  -.057  -.054  -.023  -.006  -.014  -.027;
       .000  -.010  -.022  -.034  -.047  -.060  -.069  -.067  -.033  -.036  -.035  -.035;
       .007  -.010  -.023  -.034  -.049  -.063  -.081  -.079  -.060  -.058  -.062  -.059;
       .009  -.011  -.023  -.037  -.050  -.068  -.089  -.088  -.091  -.076  -.077  -.076 ];
A = A'; 
row = 3;
col = 1;

s = 0.2 * alpha;
k = fix ( s );
if ( k <= -2 )
    k = -1;
end
if ( k >= 9 )
    k = 8;
end
da = s - k;
l = k + fix( sign ( da ) * 1.1 );
%%%%%%%%%%%%%%%%%%%%%%%%%%%%%%%%%%
% added as boundary condition
if l < -2
    l = -2;
elseif l > 9
        l = 9;
end
%%%%%%%%%%%%%%%%%%%%%%%%%%%%%%%%%%
s = 0.2 * abs( beta );
m = fix ( s );
if ( m == 0 )
   m = 1;
end
if ( m >= 6)
   m = 5;
end
db = s - m;
n = m + fix ( sign ( db ) * 1.1 );
%%%%%%%%%%%%%%%%%%%%%%%%%%%%%%%%%%
% added as boundary condition
if n < 0
    n = 0;
elseif n > 6
        n = 6;
end
%%%%%%%%%%%%%%%%%%%%%%%%%%%%%%%%%%
t = A( k+row, m+col );
u = A( k+row, n+col );
v = t + abs( da ) * ( A( l+row, m+col ) - t );
w = u + abs( da ) * ( A( l+row, n+col ) - u );
dum = v + ( w - v ) * abs( db );
cl_value = dum * sign ( beta ) * 1.0;

function cm_value = cm( alpha, el )

A = [ .205   .168   .186   .196   .213   .251   .245   .238   .252   .231   .198   .192;
      .081   .077   .107   .110   .110   .141   .127   .119   .133   .108   .081   .093;
     -.046  -.020  -.009  -.005  -.006   .010   .006  -.001   .014   .000  -.013   .032;
     -.174  -.145  -.121  -.127  -.129  -.102  -.097  -.113  -.087  -.084  -.069  -.006;
     -.259  -.202  -.184  -.193  -.199  -.150  -.160  -.167  -.104  -.076  -.041  -.005 ];
A = A';  
row = 3;
col = 3;

s = 0.2 * alpha;
k = fix ( s );
if ( k <= -2 )
    k = -1;
end
if ( k >= 9 )
    k = 8;
end
da = s - k;
l = k + fix ( sign ( da ) * 1.1 );
%%%%%%%%%%%%%%%%%%%%%%%%%%%%%%%%%%
% added as boundary condition
if l < -2
    l = -2;
elseif l > 9
        l = 9;
end
%%%%%%%%%%%%%%%%%%%%%%%%%%%%%%%%%%
s = el / 12.0;
m = fix ( s );
if ( m <= -2 )
   m = -1;
end
if ( m >= 2)
   m = 1;
end
de = s - m;
n = m + fix ( sign ( de ) * 1.1 );
%%%%%%%%%%%%%%%%%%%%%%%%%%%%%%%%%%
% added as boundary condition
if n < -2
    n = -2;
elseif n > 2
        n = 2;
end
%%%%%%%%%%%%%%%%%%%%%%%%%%%%%%%%%%
t = A( k+row, m+col );
u = A( k+row, n+col );
v = t + abs( da ) * ( A( l+row, m+col ) - t );
w = u + abs( da ) * ( A( l+row, n+col ) - u );
cm_value = v + ( w - v ) * abs( de );

function cn_value = cn( alpha, beta )

A = [ .0    .0    .0    .0    .0    .0    .0    .0    .0     .0     .0     .0  ;
      .018  .019  .018  .019  .019  .018  .013  .007  .004  -.014  -.017  -.033;
      .038  .042  .042  .042  .043  .039  .030  .017  .004  -.035  -.047  -.057;
      .056  .057  .059  .058  .058  .053  .032  .012  .002  -.046  -.071  -.073;
      .064  .077  .076  .074  .073  .057  .029  .007  .012  -.034  -.065  -.041;
      .074  .086  .093  .089  .080  .062  .049  .022  .028  -.012  -.002  -.013;
      .079  .090  .106  .106  .096  .080  .068  .030  .064   .015   .011  -.001 ];
A = A';  
row = 3;
col = 1;
  
s = 0.2 * alpha;
k = fix ( s );
if ( k <= -2 )
    k = -1;
end
if ( k >= 9 )
    k = 8;
end
da = s - k;
l = k + fix ( sign ( da ) * 1.1 );
%%%%%%%%%%%%%%%%%%%%%%%%%%%%%%%%%%
% added as boundary condition
if l < -2
    l = -2;
elseif l > 9
        l = 9;
end
%%%%%%%%%%%%%%%%%%%%%%%%%%%%%%%%%%
s = 0.2 * abs( beta );
m = fix ( s );
if ( m == 0 )
   m = 1;
end
if ( m >= 6)
   m = 5;
end
db = s - m;
n = m + fix ( sign ( db ) * 1.1 );
%%%%%%%%%%%%%%%%%%%%%%%%%%%%%%%%%%
% added as boundary condition
if n < 0
    n = 0;
elseif n > 6
        n = 6;
end
%%%%%%%%%%%%%%%%%%%%%%%%%%%%%%%%%%
t = A( k+row, m+col );
u = A( k+row, n+col );
v = t + abs( da ) * ( A( l+row, m+col ) - t );
w = u + abs( da ) * ( A( l+row, n+col ) - u );
dum = v + ( w - v ) * abs( db );
cn_value = dum * sign ( beta ) * 1.0;

function [ d ] = damping ( alpha )  

% d1 = CXq;
% d2 = CYr;
% d3 = CYp;
% d4 = CZq;
% d5 = Clr;
% d6 = Clp;
% d7 = Cmq;
% d8 = Cnr;
% d9 = Cnp;


A = [ -0.267   -0.110    0.308    1.34     2.08     2.91     2.76     2.05     1.50    1.49    1.83    1.21;
       0.882    0.852    0.876    0.958    0.962    0.974    0.819    0.483    0.590   1.21   -0.493  -1.04;
      -0.108   -0.108   -0.188    0.110    0.258    0.226    0.344    0.362    0.611   0.529   0.298  -0.227;
      -8.80    -25.8    -28.9    -31.4    -31.2    -30.7    -27.7    -28.2    -29.0   -29.8   -38.3   -35.3;
      -0.126   -0.026    0.063    0.113    0.208    0.230    0.319    0.437    0.680   0.100   0.447  -0.330;
      -0.360   -0.359   -0.443   -0.420   -0.383   -0.375   -0.329   -0.294   -0.230  -0.210  -0.120  -0.100;
      -7.21    -5.40    -5.23    -5.26    -6.11    -6.64    -5.69    -6.00    -6.20   -6.40   -6.60   -6.00;
      -0.380   -0.363   -0.378   -0.386   -0.370   -0.453   -0.550   -0.582   -0.595  -0.637  -1.02   -0.840;
       0.061    0.052    0.052   -0.012   -0.013   -0.024    0.050    0.150    0.130   0.158   0.240   0.150 ];
A = A';  
row = 3;

s = 0.2 * alpha;
k = fix ( s );
if ( k <= -2 )
    k = -1;
elseif ( k >= 9 )
    k = 8;
end
da = s - k;
l = k + fix ( sign ( da ) * 1.1 );
%%%%%%%%%%%%%%%%%%%%%%%%%%%%%%%%%%
% added as boundary condition
if l < -2
    l = -2;
elseif l > 9
        l = 9;
end
%%%%%%%%%%%%%%%%%%%%%%%%%%%%%%%%%%
d=zeros(1,9);
for ( i = 1 : 9 ) % step : i++
    d( i ) = A( k+row, i ) + abs( da ) * ( A( l+row, i ) - A( k+row, i ) );
end
d = d'; % transfer d into a column vector

== matlab function SP_linsysGet/Subsystem/sefl_built_model/Flight_dynamics/MATLAB Function ==
  data: V output; w input; u input; alpha output; w_dot input; u_dot input; alpha_dot output; V_dot output
function [V,alpha,alpha_dot,V_dot] = fcn(w,u,w_dot,u_dot)
V=400;
alpha = atan(w/u);
%V=(u^2+w^2)^0.5;
alpha_dot=(u*w_dot-w*u_dot)/V^2;
V_dot=(u*u_dot+w*w_dot)/V;

== matlab function SP_linsysGet/Subsystem/sefl_built_model/MATLAB Function2 ==
  data: W input; X output; theta input; phi input; Y output; Z output
function [X,Y,Z] = fcn(W,theta,phi)
X=-W*sin(theta);
Y=W*cos(theta)*sin(phi);
Z=W*cos(theta)*cos(phi);

== matlab function SP_linsysGet/Subsystem/sefl_built_model/dynamic head ==
  data: v input; qbar output; rho input
function qbar = fcn(v,rho)
qbar=0.5*rho*v^2;

== matlab function SP_linsysGet/Subsystem/sefl_built_model/thrust model ==
  data: pow input; thrust_value output; alt input; rmach input
function thrust_value = thrust ( pow, alt, rmach )
% A - idle
% B - military
% A - maximum

A = [  1060.0    670.0     880.0    1140.0  1500.0   1860.0; 
       635.0     425.0     690.0    1010.0  1330.0   1700.0;
        60.0     25.0      345.0     755.0  1130.0   1525.0;
      -1020.0    -710.0   -300.0     350.0   910.0   1360.0;
      -2700.0   -1900.0   -1300.0   -247.0   600.0   1100.0;
      -3600.0   -1400.0   -595.0    -342.0  -200.0    700.0 ];
A = A';  
  
B = [ 12680.0  9150.0    6200.0   3950.0   2450.0   1400.0;
      12680.0  9150.0    6313.0   4040.0   2470.0   1400.0;
      12610.0  9312.0    6610.0   4290.0   2600.0   1560.0;
      12640.0  9839.0    7090.0   4660.0   2840.0   1660.0;
      12390.0  10176.0   7750.0   5320.0   3250.0   1930.0;
      11680.0  9848.0    8050.0   6100.0   3800.0   2310.0 ];
B = B';  

C = [ 20000.0  15000.0  10800.0   7000.0   4000.0   2500.0;
      21420.0  15700.0  11225.0   7323.0   4435.0   2600.0;
      22700.0  16860.0  12250.0   8154.0   5000.0   2835.0;
      24240.0  18910.0  13760.0   9285.0   5700.0   3215.0;
      26070.0  21075.0  15975.0  11115.0   6860.0   3950.0;
      28886.0  23319.0  18300.0  13484.0   8642.0   5057.0 ];  
C = C';  

row = 1;
col = 1;

h = 0.0001 * alt;
i = fix( h );
if (i >= 5)
    i = 4;
elseif (i <= 0)
     i = 0;
end
dh = h - i;
rm = 5.0 * rmach;
%  disp('rmach'); rmach
m = fix( rm );
if ( m >= 5 )
    m = 4;
elseif (m <= 0)
     m = 0;
end
dm = rm - m;
cdh = 1.0 - dh;
%  disp('i+row'); i+row
%  disp('m+row'); m+row
s = B( i+row, m+col ) * cdh + B( i+1+row, m+col ) * dh;
t = B( i+row, m+1+col ) * cdh + B( i+1+row, m+1+col ) * dh;
tmil = s + ( t - s ) * dm;
if( pow < 50.0 )
    s = A( i+row, m+col )   * cdh + A( i+1+row, m+col ) * dh;
    t = A( i+row, m+1+col ) * cdh + A( i+1+row, m+1+col ) * dh;
    tidl = s + ( t - s ) * dm;
    thrust_value = tidl + ( tmil - tidl ) * pow *0.02;
else
    s = C( i+row, m+col )   * cdh + C( i+1+row, m+col ) * dh;
    t = C( i+row, m+1+col ) * cdh + C( i+1+row, m+1+col ) * dh;
    tmax = s + ( t - s ) * dm;
    thrust_value = tmil + ( tmax - tmil ) * ( pow - 50.0 ) * 0.02;
end
